simulink model "asiaa_adc5g"  (R2016b)
settings: Solver=VariableStepAuto  StartTime=0.0  StopTime=10.0  RelTol=1e-3
libraries: xbsIndex_r4 x17
settings Model: Creator=qwerty40  LastModifiedBy=qwerty40

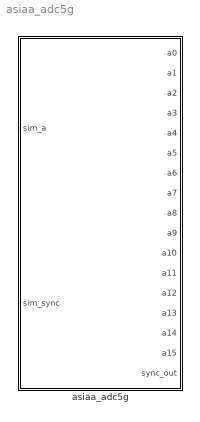
== system asiaa_adc5g ==
  asiaa_adc5g : Subsystem  Tag=xps:adc5g  mask(adc5g){input_mode=One-channel -- A, adc_brd=ZDOK 0, demux=1:2, adc_bit_width=4, adc_clk_rate=2500, using_ctrl=on, test_ramp=off}
      mask prompts: input_mode "Input mode:"; adc_brd "ADC Board"; demux "Internal demux"; adc_bit_width "ADC Resolution (bits):"; adc_clk_rate "ADC Clock Rate (MHz):"; using_ctrl "use control"; test_ramp "start in test ramp mode"
      mask help:
      | Interface for the ASIAA 5 GSps ADC. Supports interleaving all four
      | cores using either input A or C, or interleaving two-cores each for
      | A and C. The hardware itself comes in two versions:
      |
      | DMUX 1:2 -- 4-bit samples, 4 parallel streams
      | DMUX 1:1 -- 8-bit samples, 2 parallel streams
      |
      | In either configuration this block will output 8 parallel streams
      | but the underlying interface, and the bitwidth of the samples,
      | will be different.
      mask init:
      | adc5g_init(gcb,...
      |     'input_mode', input_mode,...
      |     'demux', demux,...
      |     'adc_clk_rate', adc_clk_rate,...
      |     'adc_bit_width', adc_bit_width,...
      |     'adc_brd', adc_brd,...
      |     'using_ctrl', using_ctrl,...
      |     'test_ramp', test_ramp);
      mask TypeOptions input_mode: One-channel -- A | One-channel -- C | Two-channel -- A&C
      mask TypeOptions adc_brd: ZDOK 0 | ZDOK 1
      mask TypeOptions demux: 1:1 | 1:2
      mask Callback demux:
      | demux = get_param(gcb,'demux');
      | if(strcmp(demux,'1:1')),
      |     set_param(gcb, 'adc_bit_width', '8')
      | elseif(strcmp(demux, '1:2')),
      |     set_param(gcb, 'adc_bit_width', '4');
      | else
      | end

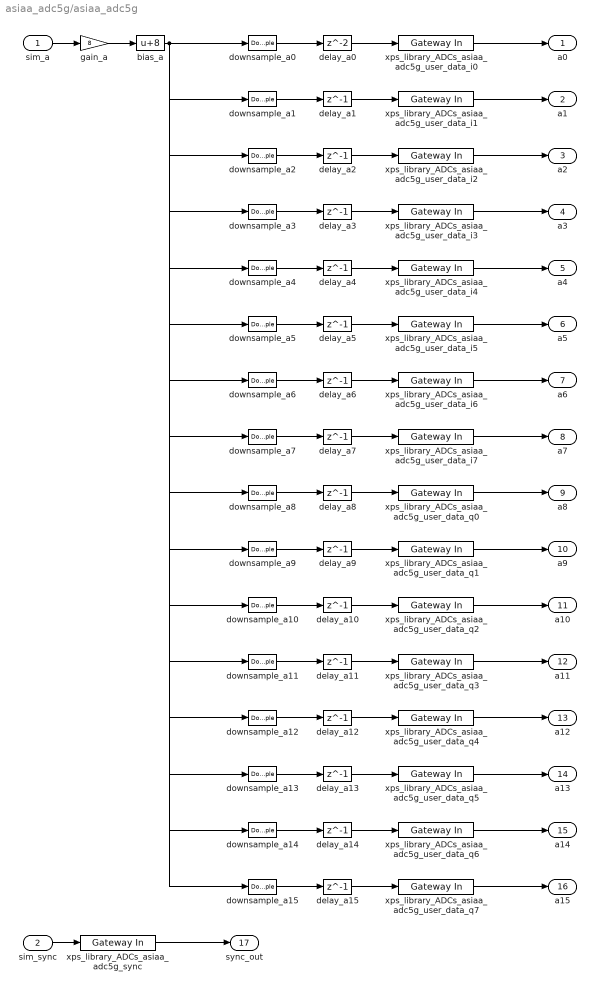
== system asiaa_adc5g/asiaa_adc5g ==
  sim_a : Inport
  sim_sync : Inport  Port=2
  bias_a : Bias  Bias=8  SaturateOnIntegerOverflow=on
  delay_a0 : Delay  InitialCondition=0  InputProcessing=Inherited
  delay_a{1..15} (15 alike) : Delay  DelayLength=1  InitialCondition=0  InputProcessing=Inherited
  downsample_a0 : DownSample  N=16  RateOptions=Allow multirate processing
  downsample_a1 : DownSample  N=16  phase=1  RateOptions=Allow multirate processing
  downsample_a10 : DownSample  N=16  phase=10  RateOptions=Allow multirate processing
  downsample_a11 : DownSample  N=16  phase=11  RateOptions=Allow multirate processing
  downsample_a12 : DownSample  N=16  phase=12  RateOptions=Allow multirate processing
  downsample_a13 : DownSample  N=16  phase=13  RateOptions=Allow multirate processing
  downsample_a14 : DownSample  N=16  phase=14  RateOptions=Allow multirate processing
  downsample_a15 : DownSample  N=16  phase=15  RateOptions=Allow multirate processing
  downsample_a2 : DownSample  N=16  phase=2  RateOptions=Allow multirate processing
  downsample_a3 : DownSample  N=16  phase=3  RateOptions=Allow multirate processing
  downsample_a4 : DownSample  N=16  phase=4  RateOptions=Allow multirate processing
  downsample_a5 : DownSample  N=16  phase=5  RateOptions=Allow multirate processing
  downsample_a6 : DownSample  N=16  phase=6  RateOptions=Allow multirate processing
  downsample_a7 : DownSample  N=16  phase=7  RateOptions=Allow multirate processing
  downsample_a8 : DownSample  N=16  phase=8  RateOptions=Allow multirate processing
  downsample_a9 : DownSample  N=16  phase=9  RateOptions=Allow multirate processing
  gain_a : Gain  Gain=8  SaturateOnIntegerOverflow=on  OutDataTypeStr=Inherit: Same as input  ParamDataTypeStr=Inherit: Same as input
  xps_library_ADCs_asiaa_adc5g_sync : xbsIndex_r4/Gateway In  gui_display_data_type=Fixed-point  arith_type=Boolean  n_bits=16  bin_pt=14  preci_type=Single  exp_width=8  frac_width=24  rows=1  columns=1  quantization="Round  (unbiased: +/- Inf)"  overflow=Saturate  period=1  UseAsADC=off  ADCChannel='1'  interface=None  automatic_assignment=on  address_offset=hex2dec('00')  intf_name=''  intf_description=''  default_value=0  timing_constraint=None  locs_specified=off  LOCs={}  io_standard={}  inherit_from_input=off  hdl_port=on  dbl_ovrd=off  block_type=gatewayin
  xps_library_ADCs_asiaa_adc5g_user_data_i{0..7} (8 alike) : xbsIndex_r4/Gateway In  gui_display_data_type=Fixed-point  arith_type=Unsigned  n_bits=4  bin_pt=0  preci_type=Single  exp_width=8  frac_width=24  rows=1  columns=1  quantization=Truncate  overflow=Wrap  period=1  UseAsADC=off  ADCChannel='1'  interface=None  automatic_assignment=on  address_offset=hex2dec('00')  intf_name=''  intf_description=''  default_value=0  timing_constraint=None  locs_specified=off  LOCs={}  io_standard={}  inherit_from_input=off  hdl_port=on  dbl_ovrd=off  block_type=gatewayin
  xps_library_ADCs_asiaa_adc5g_user_data_q{0..7} (8 alike) : xbsIndex_r4/Gateway In  gui_display_data_type=Fixed-point  arith_type=Unsigned  n_bits=4  bin_pt=0  preci_type=Single  exp_width=8  frac_width=24  rows=1  columns=1  quantization=Truncate  overflow=Wrap  period=1  UseAsADC=off  ADCChannel='1'  interface=None  automatic_assignment=on  address_offset=hex2dec('00')  intf_name=''  intf_description=''  default_value=0  timing_constraint=None  locs_specified=off  LOCs={}  io_standard={}  inherit_from_input=off  hdl_port=on  dbl_ovrd=off  block_type=gatewayin
  a0 : Outport
  a1 : Outport  Port=2
  a2 : Outport  Port=3
  a3 : Outport  Port=4
  a4 : Outport  Port=5
  a5 : Outport  Port=6
  a6 : Outport  Port=7
  a7 : Outport  Port=8
  a8 : Outport  Port=9
  a9 : Outport  Port=10
  a10 : Outport  Port=11
  a11 : Outport  Port=12
  a12 : Outport  Port=13
  a13 : Outport  Port=14
  a14 : Outport  Port=15
  a15 : Outport  Port=16
  sync_out : Outport  Port=17
  wires:
  xps_library_ADCs_asiaa_adc5g_sync/1 -> sync_out/1
  sim_sync/1 -> xps_library_ADCs_asiaa_adc5g_sync/1
  xps_library_ADCs_asiaa_adc5g_user_data_q7/1 -> a15/1
  delay_a15/1 -> xps_library_ADCs_asiaa_adc5g_user_data_q7/1
  downsample_a15/1 -> delay_a15/1
  xps_library_ADCs_asiaa_adc5g_user_data_q6/1 -> a14/1
  delay_a14/1 -> xps_library_ADCs_asiaa_adc5g_user_data_q6/1
  downsample_a14/1 -> delay_a14/1
  xps_library_ADCs_asiaa_adc5g_user_data_q5/1 -> a13/1
  delay_a13/1 -> xps_library_ADCs_asiaa_adc5g_user_data_q5/1
  downsample_a13/1 -> delay_a13/1
  xps_library_ADCs_asiaa_adc5g_user_data_q4/1 -> a12/1
  delay_a12/1 -> xps_library_ADCs_asiaa_adc5g_user_data_q4/1
  downsample_a12/1 -> delay_a12/1
  xps_library_ADCs_asiaa_adc5g_user_data_q3/1 -> a11/1
  delay_a11/1 -> xps_library_ADCs_asiaa_adc5g_user_data_q3/1
  downsample_a11/1 -> delay_a11/1
  xps_library_ADCs_asiaa_adc5g_user_data_q2/1 -> a10/1
  delay_a10/1 -> xps_library_ADCs_asiaa_adc5g_user_data_q2/1
  downsample_a10/1 -> delay_a10/1
  xps_library_ADCs_asiaa_adc5g_user_data_q1/1 -> a9/1
  delay_a9/1 -> xps_library_ADCs_asiaa_adc5g_user_data_q1/1
  downsample_a9/1 -> delay_a9/1
  xps_library_ADCs_asiaa_adc5g_user_data_q0/1 -> a8/1
  delay_a8/1 -> xps_library_ADCs_asiaa_adc5g_user_data_q0/1
  downsample_a8/1 -> delay_a8/1
  xps_library_ADCs_asiaa_adc5g_user_data_i7/1 -> a7/1
  delay_a7/1 -> xps_library_ADCs_asiaa_adc5g_user_data_i7/1
  downsample_a7/1 -> delay_a7/1
  xps_library_ADCs_asiaa_adc5g_user_data_i6/1 -> a6/1
  delay_a6/1 -> xps_library_ADCs_asiaa_adc5g_user_data_i6/1
  downsample_a6/1 -> delay_a6/1
  xps_library_ADCs_asiaa_adc5g_user_data_i5/1 -> a5/1
  delay_a5/1 -> xps_library_ADCs_asiaa_adc5g_user_data_i5/1
  downsample_a5/1 -> delay_a5/1
  xps_library_ADCs_asiaa_adc5g_user_data_i4/1 -> a4/1
  delay_a4/1 -> xps_library_ADCs_asiaa_adc5g_user_data_i4/1
  downsample_a4/1 -> delay_a4/1
  xps_library_ADCs_asiaa_adc5g_user_data_i3/1 -> a3/1
  delay_a3/1 -> xps_library_ADCs_asiaa_adc5g_user_data_i3/1
  downsample_a3/1 -> delay_a3/1
  xps_library_ADCs_asiaa_adc5g_user_data_i2/1 -> a2/1
  delay_a2/1 -> xps_library_ADCs_asiaa_adc5g_user_data_i2/1
  downsample_a2/1 -> delay_a2/1
  xps_library_ADCs_asiaa_adc5g_user_data_i1/1 -> a1/1
  delay_a1/1 -> xps_library_ADCs_asiaa_adc5g_user_data_i1/1
  downsample_a1/1 -> delay_a1/1
  xps_library_ADCs_asiaa_adc5g_user_data_i0/1 -> a0/1
  delay_a0/1 -> xps_library_ADCs_asiaa_adc5g_user_data_i0/1
  downsample_a0/1 -> delay_a0/1
  bias_a/1 -> downsample_a15/1, downsample_a14/1, downsample_a13/1, downsample_a12/1, downsample_a11/1, downsample_a10/1, downsample_a9/1, downsample_a8/1, downsample_a7/1, downsample_a6/1, downsample_a5/1, downsample_a4/1, downsample_a3/1, downsample_a2/1, downsample_a1/1, downsample_a0/1
  gain_a/1 -> bias_a/1
  sim_a/1 -> gain_a/1
